simulink model "h16k_ver110_1080"  (R2012b)
settings: Solver=VariableStepDiscrete  SolverMode=SingleTasking  StartTime=0.0  StopTime=128000  RelTol=1e-3
undefined symbols (not defined in the file or in its folder): sfp
libraries: xbsIndex_r4 x3384, dspsigops x32, casper_library_misc x23, monroe_library x8, simulink x7, xps_library x6
(part 6 of 28)

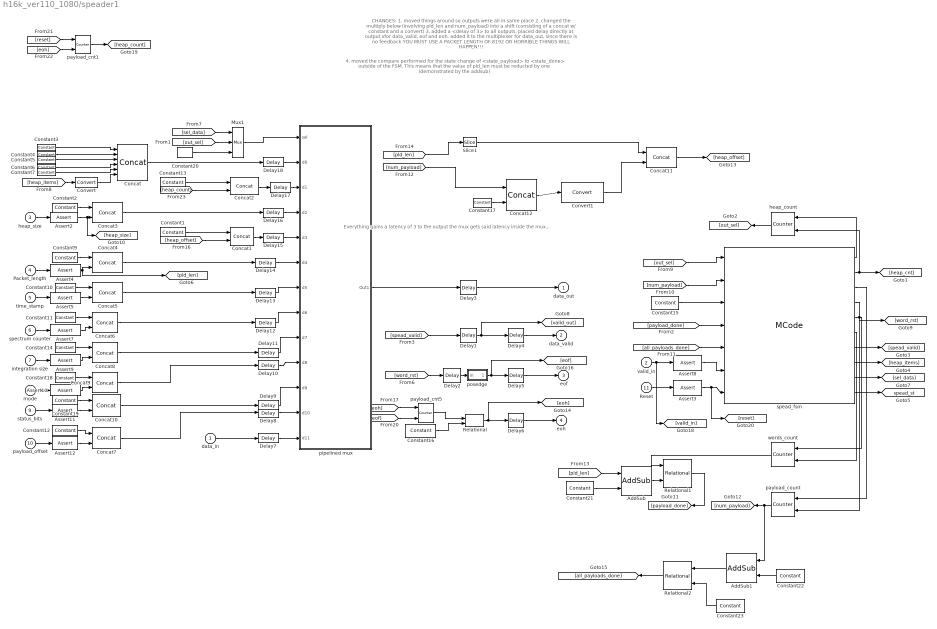
== system h16k_ver110_1080/speader1 ==
  note: Everything gains a latency of 3 to the output
      | the mux gets said latency inside the mux...
  note: CHANGES:
      | 1. moved things around so outputs were all in same place
      | 2. changed the multiply below (involving pld_len and num_payload) into a shift (consisting of a concat w/ constant and a convert)
      | 3. added a <delay of 3> to all outputs.  placed delay directly at output vfor data_valid, eof and eoh.  added it to the multiplexer for data_out, since there is no feedback
      |
      | YOU MUST USE A PACKET LENGTH OF 8192 OR HORRIBLE THINGS WILL HAPPEN!!!
  note: 4. moved the compare performed for the state change of <state_oayload> to <state_done> outside of the FSM.
      | This means that the value of pld_len must be reducted by one (demonstrated by the addsub)
  data_in : Inport
  valid_in : Inport  Port=2
  heap_size : Inport  Port=3
  Packet_length : Inport  Port=4
  time_stamp : Inport  Port=5
  spectrum counter : Inport  Port=6
  integration size : Inport  Port=7
  mode : Inport  Port=8
  status_bits : Inport  Port=9
  payload_offset : Inport  Port=10
  Reset : Inport  Port=11
  AddSub : xbsIndex_r4/AddSub  mode=Subtraction  use_carryin=off  use_carryout=off  en=off  latency=0  precision=User Defined  arith_type=Unsigned  n_bits=40  bin_pt=0  quantization=Truncate  overflow=Wrap  dbl_ovrd=off  use_behavioral_HDL=off  hw_selection=Fabric  pipelined=off  block_type=addsub
  AddSub1 : xbsIndex_r4/AddSub  mode=Addition  use_carryin=off  use_carryout=off  en=off  latency=1  precision=User Defined  arith_type=Unsigned  n_bits=8  bin_pt=0  quantization=Truncate  overflow=Wrap  dbl_ovrd=off  use_behavioral_HDL=off  hw_selection=Fabric  pipelined=off  block_type=addsub
  Assert{2,4..5,7,9..12} (8 alike) : xbsIndex_r4/Assert  assert_type=on  type_source=Explicitly  gui_display_data_type=Fixed-point  arith_type=Unsigned  n_bits=spead_lsw  bin_pt=0  preci_type=Single  exp_width=8  frac_width=24  assert_rate=off  rate_source=Explicitly  period=1  output_port=on  block_type=assert
      settings: block_version=11.4
  Assert3 : xbsIndex_r4/Assert  assert_type=on  type_source=Explicitly  gui_display_data_type=Fixed-point  arith_type=Boolean  n_bits=spead_lsw  bin_pt=0  preci_type=Single  exp_width=8  frac_width=24  assert_rate=on  rate_source=Explicitly  period=1  output_port=on  block_type=assert
      settings: block_version=11.4
  Assert8 : xbsIndex_r4/Assert  assert_type=on  type_source=Explicitly  gui_display_data_type=Fixed-point  arith_type=Boolean  n_bits=spead_lsw  bin_pt=0  preci_type=Single  exp_width=8  frac_width=24  assert_rate=on  rate_source=Explicitly  period=1  output_port=on  block_type=assert
      settings: block_version=11.4
  Concat : xbsIndex_r4/Concat  num_inputs=6  dbl_ovrd=off  block_type=concat
  Concat{1..12} (12 alike) : xbsIndex_r4/Concat  num_inputs=2  dbl_ovrd=off  block_type=concat
  Constant1 : xbsIndex_r4/Constant  const=8388608+3  gui_display_data_type=Fixed-point  arith_type=Unsigned  n_bits=spead_msw-spead_lsw  bin_pt=0  preci_type=Single  exp_width=8  frac_width=24  explicit_period=on  period=1  equ=P=C  opselect=C  inp2=PCIN>>17  opr=+  inp1=P  carry=CIN  dbl_ovrd=off  block_type=constant
      settings: block_version=11.4
  Constant10 : xbsIndex_r4/Constant  const=8388608+32  gui_display_data_type=Fixed-point  arith_type=Unsigned  n_bits=spead_msw-spead_lsw  bin_pt=0  preci_type=Single  exp_width=8  frac_width=24  explicit_period=on  period=1  equ=P=C  opselect=C  inp2=PCIN>>17  opr=+  inp1=P  carry=CIN  dbl_ovrd=off  block_type=constant
      settings: block_version=11.4
  Constant11 : xbsIndex_r4/Constant  const=8388608+33  gui_display_data_type=Fixed-point  arith_type=Unsigned  n_bits=spead_msw-spead_lsw  bin_pt=0  preci_type=Single  exp_width=8  frac_width=24  explicit_period=on  period=1  equ=P=C  opselect=C  inp2=PCIN>>17  opr=+  inp1=P  carry=CIN  dbl_ovrd=off  block_type=constant
      settings: block_version=11.4
  Constant12 : xbsIndex_r4/Constant  const=37  gui_display_data_type=Fixed-point  arith_type=Unsigned  n_bits=spead_msw-spead_lsw  bin_pt=0  preci_type=Single  exp_width=8  frac_width=24  explicit_period=on  period=1  equ=P=C  opselect=C  inp2=PCIN>>17  opr=+  inp1=P  carry=CIN  dbl_ovrd=off  block_type=constant
      settings: block_version=11.4
  Constant13 : xbsIndex_r4/Constant  const=8388608+1  gui_display_data_type=Fixed-point  arith_type=Unsigned  n_bits=spead_msw-spead_lsw  bin_pt=0  preci_type=Single  exp_width=8  frac_width=24  explicit_period=on  period=1  equ=P=C  opselect=C  inp2=PCIN>>17  opr=+  inp1=P  carry=CIN  dbl_ovrd=off  block_type=constant
      settings: block_version=11.4
  Constant14 : xbsIndex_r4/Constant  const=8388608+34  gui_display_data_type=Fixed-point  arith_type=Unsigned  n_bits=spead_msw-spead_lsw  bin_pt=0  preci_type=Single  exp_width=8  frac_width=24  explicit_period=on  period=1  equ=P=C  opselect=C  inp2=PCIN>>17  opr=+  inp1=P  carry=CIN  dbl_ovrd=off  block_type=constant
      settings: block_version=11.4
  Constant15 : xbsIndex_r4/Constant  const=num_items+5  gui_display_data_type=Fixed-point  arith_type=Unsigned  n_bits=8  bin_pt=0  preci_type=Single  exp_width=8  frac_width=24  explicit_period=on  period=1  equ=P=C  opselect=C  inp2=PCIN>>17  opr=+  inp1=P  carry=CIN  dbl_ovrd=off  block_type=constant
      settings: block_version=11.4
  Constant16 : xbsIndex_r4/Constant  const=num_payloads  gui_display_data_type=Fixed-point  arith_type=Unsigned  n_bits=16  bin_pt=0  preci_type=Single  exp_width=8  frac_width=24  explicit_period=on  period=1  equ=P=C  opselect=C  inp2=PCIN>>17  opr=+  inp1=P  carry=CIN  dbl_ovrd=off  block_type=constant
      settings: block_version=11.4
  Constant17 : xbsIndex_r4/Constant  const=0  gui_display_data_type=Fixed-point  arith_type=Unsigned  n_bits=13  bin_pt=0  preci_type=Single  exp_width=8  frac_width=24  explicit_period=on  period=1  equ=P=C  opselect=C  inp2=PCIN>>17  opr=+  inp1=P  carry=CIN  dbl_ovrd=off  block_type=constant
  Constant18 : xbsIndex_r4/Constant  const=8388608+35  gui_display_data_type=Fixed-point  arith_type=Unsigned  n_bits=spead_msw-spead_lsw  bin_pt=0  preci_type=Single  exp_width=8  frac_width=24  explicit_period=on  period=1  equ=P=C  opselect=C  inp2=PCIN>>17  opr=+  inp1=P  carry=CIN  dbl_ovrd=off  block_type=constant
      settings: block_version=11.4
  Constant19 : xbsIndex_r4/Constant  const=8388608+36  gui_display_data_type=Fixed-point  arith_type=Unsigned  n_bits=spead_msw-spead_lsw  bin_pt=0  preci_type=Single  exp_width=8  frac_width=24  explicit_period=on  period=1  equ=P=C  opselect=C  inp2=PCIN>>17  opr=+  inp1=P  carry=CIN  dbl_ovrd=off  block_type=constant
      settings: block_version=11.4
  Constant2 : xbsIndex_r4/Constant  const=8388608+2  gui_display_data_type=Fixed-point  arith_type=Unsigned  n_bits=spead_msw-spead_lsw  bin_pt=0  preci_type=Single  exp_width=8  frac_width=24  explicit_period=on  period=1  equ=P=C  opselect=C  inp2=PCIN>>17  opr=+  inp1=P  carry=CIN  dbl_ovrd=off  block_type=constant
      settings: block_version=11.4
  Constant20 : xbsIndex_r4/Constant  const=num_items+5  gui_display_data_type=Fixed-point  arith_type=Unsigned  n_bits=4  bin_pt=0  preci_type=Single  exp_width=8  frac_width=24  explicit_period=on  period=1  equ=P=C  opselect=C  inp2=PCIN>>17  opr=+  inp1=P  carry=CIN  dbl_ovrd=off  block_type=constant
      settings: block_version=11.4
  Constant21 : xbsIndex_r4/Constant  const=8  gui_display_data_type=Fixed-point  arith_type=Unsigned  n_bits=4  bin_pt=0  preci_type=Single  exp_width=8  frac_width=24  explicit_period=on  period=1  equ=P=C  opselect=C  inp2=PCIN>>17  opr=+  inp1=P  carry=CIN  dbl_ovrd=off  block_type=constant
      settings: block_version=11.4
  Constant22 : xbsIndex_r4/Constant  const=1  gui_display_data_type=Fixed-point  arith_type=Unsigned  n_bits=1  bin_pt=0  preci_type=Single  exp_width=8  frac_width=24  explicit_period=on  period=1  equ=P=C  opselect=C  inp2=PCIN>>17  opr=+  inp1=P  carry=CIN  dbl_ovrd=off  block_type=constant
      settings: block_version=11.4
  Constant23 : xbsIndex_r4/Constant  const=num_payloads  gui_display_data_type=Fixed-point  arith_type=Unsigned  n_bits=8  bin_pt=0  preci_type=Single  exp_width=8  frac_width=24  explicit_period=on  period=1  equ=P=C  opselect=C  inp2=PCIN>>17  opr=+  inp1=P  carry=CIN  dbl_ovrd=off  block_type=constant
      settings: block_version=11.4
  Constant3 : xbsIndex_r4/Constant  const=83  gui_display_data_type=Fixed-point  arith_type=Unsigned  n_bits=8  bin_pt=0  preci_type=Single  exp_width=8  frac_width=24  explicit_period=on  period=1  equ=P=C  opselect=C  inp2=PCIN>>17  opr=+  inp1=P  carry=CIN  dbl_ovrd=off  block_type=constant
      settings: block_version=11.4
  Constant4 : xbsIndex_r4/Constant  const=4  gui_display_data_type=Fixed-point  arith_type=Unsigned  n_bits=8  bin_pt=0  preci_type=Single  exp_width=8  frac_width=24  explicit_period=on  period=1  equ=P=C  opselect=C  inp2=PCIN>>17  opr=+  inp1=P  carry=CIN  dbl_ovrd=off  block_type=constant
      settings: block_version=11.4
  Constant5 : xbsIndex_r4/Constant  const=3  gui_display_data_type=Fixed-point  arith_type=Unsigned  n_bits=8  bin_pt=0  preci_type=Single  exp_width=8  frac_width=24  explicit_period=on  period=1  equ=P=C  opselect=C  inp2=PCIN>>17  opr=+  inp1=P  carry=CIN  dbl_ovrd=off  block_type=constant
      settings: block_version=11.4
  Constant6 : xbsIndex_r4/Constant  const=5  gui_display_data_type=Fixed-point  arith_type=Unsigned  n_bits=8  bin_pt=0  preci_type=Single  exp_width=8  frac_width=24  explicit_period=on  period=1  equ=P=C  opselect=C  inp2=PCIN>>17  opr=+  inp1=P  carry=CIN  dbl_ovrd=off  block_type=constant
      settings: block_version=11.4
  Constant7 : xbsIndex_r4/Constant  const=0  gui_display_data_type=Fixed-point  arith_type=Unsigned  n_bits=16  bin_pt=0  preci_type=Single  exp_width=8  frac_width=24  explicit_period=on  period=1  equ=P=C  opselect=C  inp2=PCIN>>17  opr=+  inp1=P  carry=CIN  dbl_ovrd=off  block_type=constant
      settings: block_version=11.4
  Constant9 : xbsIndex_r4/Constant  const=8388608+4  gui_display_data_type=Fixed-point  arith_type=Unsigned  n_bits=spead_msw-spead_lsw  bin_pt=0  preci_type=Single  exp_width=8  frac_width=24  explicit_period=on  period=1  equ=P=C  opselect=C  inp2=PCIN>>17  opr=+  inp1=P  carry=CIN  dbl_ovrd=off  block_type=constant
      settings: block_version=11.4
  Convert : xbsIndex_r4/Convert  gui_display_data_type=Fixed-point  arith_type=Unsigned  n_bits=16  bin_pt=0  float_type=Single  exp_bits=8  fraction_bits=24  quantization=Truncate  overflow=Wrap  en=off  latency=0  dbl_ovrd=off  pipeline=off  block_type=convert
      settings: block_version=11.4
  Convert1 : xbsIndex_r4/Convert  gui_display_data_type=Fixed-point  arith_type=Unsigned  n_bits=25  bin_pt=0  float_type=Single  exp_bits=8  fraction_bits=24  quantization=Truncate  overflow=Wrap  en=off  latency=3  dbl_ovrd=off  pipeline=off  block_type=convert
  Delay{1,3,7..18} (14 alike) : xbsIndex_r4/Delay  rst=off  infoeditControl=Selection of Reset will increase slice count due to use of real FFs and instead of SRLs  en=off  latency=1  dbl_ovrd=off  reg_retiming=on  block_type=delay
      settings: block_version=11.4
  Delay2 : xbsIndex_r4/Delay  rst=off  infoeditControl=Selection of Reset will increase slice count due to use of real FFs and instead of SRLs  en=off  latency=0  dbl_ovrd=off  reg_retiming=on  block_type=delay
      settings: block_version=11.4
  Delay4 : xbsIndex_r4/Delay  rst=off  infoeditControl=Selection of Reset will increase slice count due to use of real FFs and instead of SRLs  en=off  latency=3  dbl_ovrd=off  reg_retiming=on  block_type=delay
      settings: block_version=11.4
  Delay5 : xbsIndex_r4/Delay  rst=off  infoeditControl=Selection of Reset will increase slice count due to use of real FFs and instead of SRLs  en=off  latency=3  dbl_ovrd=off  reg_retiming=on  block_type=delay
      settings: block_version=11.4
  Delay6 : xbsIndex_r4/Delay  rst=off  infoeditControl=Selection of Reset will increase slice count due to use of real FFs and instead of SRLs  en=off  latency=3  dbl_ovrd=off  reg_retiming=on  block_type=delay
      settings: block_version=11.4
  Mux1 : xbsIndex_r4/Mux  inputs=2  en=off  latency=1  precision=Full  arith_type="Signed  (2's comp)"  n_bits=8  bin_pt=2  quantization=Truncate  overflow=Wrap  dbl_ovrd=off  block_type=mux
      settings: block_version=11.4
  Relational : xbsIndex_r4/Relational  mode=a=b  en=off  latency=0  dbl_ovrd=off  block_type=relational
  Relational1 : xbsIndex_r4/Relational  mode=a=b  en=off  latency=1  dbl_ovrd=off  block_type=relational
  Relational2 : xbsIndex_r4/Relational  mode=a=b  en=off  latency=1  dbl_ovrd=off  block_type=relational
  Slice1 : xbsIndex_r4/Slice  nbits=15  boolean_output=off  mode=Upper Bit Location + Width  bit1=0  base1=MSB of Input  bit0=0  base0=LSB of Input  dbl_ovrd=off  block_type=slice
      settings: block_version=10.1.3
  heap_count : xbsIndex_r4/Counter  cnt_type=Free Running  cnt_to=Inf  operation=Up  start_count=0  cnt_by_val=1  arith_type=Unsigned  n_bits=4  bin_pt=0  load_pin=off  rst=on  en=on  explicit_period=on  period=1  dbl_ovrd=off  use_behavioral_HDL=off  implementation=Fabric  block_type=counter
      settings: block_version=11.4
  payload_cnt1 : xbsIndex_r4/Counter  cnt_type=Free Running  cnt_to=0  operation=Up  start_count=1024  cnt_by_val=1  arith_type=Unsigned  n_bits=40  bin_pt=0  load_pin=off  rst=on  en=on  explicit_period=on  period=1  dbl_ovrd=off  use_behavioral_HDL=off  implementation=Fabric  use_rpm=on  block_type=counter
      settings: xl_area=[0, 0, 0, 0, 0, 0, 0]
  payload_cnt5 : xbsIndex_r4/Counter  cnt_type=Free Running  cnt_to=0  operation=Up  start_count=0  cnt_by_val=1  arith_type=Unsigned  n_bits=16  bin_pt=0  load_pin=off  rst=on  en=on  explicit_period=on  period=1  dbl_ovrd=off  use_behavioral_HDL=off  implementation=Fabric  use_rpm=on  block_type=counter
      settings: xl_area=[0, 0, 0, 0, 0, 0, 0]
  payload_count : xbsIndex_r4/Counter  cnt_type=Free Running  cnt_to=Inf  operation=Up  start_count=0  cnt_by_val=1  arith_type=Unsigned  n_bits=8  bin_pt=0  load_pin=off  rst=on  en=on  explicit_period=on  period=1  dbl_ovrd=off  use_behavioral_HDL=off  implementation=Fabric  block_type=counter
      settings: block_version=11.4
  pipelined mux : Subsystem
  posedge : Subsystem  AncestorBlock=casper_library_misc/edge_detect  mask(edge_detect){edge=Rising, polarity=Active High, x_in=[0 0.08 0.08 0.16 0.16 0.24 0.24 0.32 0.32 0.4], y_in=[-1 -1  1  1  1  1  1  1  1  1], x_out=[0.6 0.68 0.68 0.76 0.76 0.84 0.84 0.92 0.92 1], y_out=[-1 -1  1  1 -1 -1 -1 -1 -1 -1]}
      mask prompts: edge "Edge Type"; polarity "Output Polarity"; x_in "Input X Positions"; y_in "Input Y Positions"; x_out "Output X Positions"; y_out "Output Y Positions"
      mask help: Output is active for one-cycle after each edge of the specified type (i.e. rising, falling or both).
      mask init: same as h16k_ver110_1080/edge_detect
      settings: AttributesFormatString=|
      | rising edges
      | active high
      mask Help: Output is active for one-cycle after each edge of the specified type (i.e. rising, falling, or both).  Latency is zero.
      mask TypeOptions edge: Rising | Falling | Both
      mask TypeOptions polarity: Active High | Active Low
      mask Display:
      | plot(x_in_num,0.5+y_in_num*0.2);
      | plot(x_out_num,0.5+y_out_num*0.2);
  spead_fsm : xbsIndex_r4/MCode  mfname=spead_fsm_v2  explicit_period=on  period=1  inputsTable={'boundInpExpr'=>['','','','5','','','',''],'inputs'=>['head_count','num_payload_sent','total_header_len','min_header_len','payload_done','all_payloads_done','data_valid_in','rst']}  outputsTable={'outputs'=>['head_count_rst','head_count_en','num_payload_rst','num_payload_en','words_sent_rst','words_sent_en','tge_valid','heap_elements','select_data','st'],'suppressOut'=>['off','off','off','off','off','off','off','off','off','off']}  dbl_ovrd=off  enable_stdout=off  enable_debug=off  suppress_output=on  defparams={'min_header_len',5}  hide_port_list={}  block_type=mcode
      settings: block_version=11.4
  words_count : xbsIndex_r4/Counter  cnt_type=Free Running  cnt_to=Inf  operation=Up  start_count=0  cnt_by_val=8  arith_type=Unsigned  n_bits=15  bin_pt=0  load_pin=off  rst=on  en=on  explicit_period=on  period=1  dbl_ovrd=off  use_behavioral_HDL=off  implementation=Fabric  block_type=counter
      settings: block_version=11.4
  data_out : Outport
  data_valid : Outport  Port=2
  eof : Outport  Port=3
  eoh : Outport  Port=4
  tag scope: spead_st=global
  wires:
  Slice1/1 -> Concat11/1
  Concat11/1 -> [heap_offset]
  [eoh] -> payload_cnt1/2
  [reset] -> payload_cnt1/1
  payload_cnt1/1 -> [heap_count]
  payload_cnt5/1 -> Relational/1
  Constant16/1 -> Relational/2
  Relational/1 -> [eoh], Delay6/1
  [eof] -> payload_cnt5/2
  [eoh] -> payload_cnt5/1
  [sel_data] -> Mux1/1
  [out_sel] -> Mux1/2
  pipelined mux/1(Out1) -> Delay3/1
  [pld_len] -> Slice1/1
  [num_payload] -> Concat12/1
  Delay2/1 -> posedge/1(in)
  Constant15/1 -> spead_fsm/3
  [all_payloads_done] -> spead_fsm/5
  Assert8/1 -> spead_fsm/6
  Assert3/1 -> [reset], spead_fsm/7
  [word_rst] -> Delay2/1
  posedge/1(out) -> [eof], Delay5/1
  [num_payload] -> spead_fsm/2
  [out_sel] -> spead_fsm/1
  heap_count/1 -> [out_sel]
  payload_count/1 -> [num_payload], AddSub1/1
  Convert/1 -> Concat/6
  [heap_items] -> Convert/1
  spead_fsm/9 -> [sel_data]
  spead_fsm/10 -> [spead_st]
  Mux1/1 -> pipelined mux/1(sel)
  Constant20/1 -> Mux1/3
  Reset/1 -> Assert3/1
  [heap_offset] -> Concat1/2
  valid_in/1 -> [valid_in], Assert8/1
  spead_fsm/8 -> [heap_items]
  spead_fsm/7 -> [spead_valid]
  spead_fsm/2 -> [heap_cnt], heap_count/2
  spead_fsm/1 -> heap_count/1
  spead_fsm/4 -> [word_rst], payload_count/2
  spead_fsm/3 -> payload_count/1
  spead_fsm/6 -> words_count/2
  spead_fsm/5 -> words_count/1
  Concat8/1 -> Delay11/1
  Constant14/1 -> Concat8/1
  Assert9/1 -> Concat8/2
  integration size/1 -> Assert9/1
  Concat5/1 -> Delay13/1
  Concat6/1 -> Delay12/1
  Constant11/1 -> Concat6/1
  Assert7/1 -> Concat6/2
  spectrum counter/1 -> Assert7/1
  Concat9/1 -> Delay10/1
  Concat10/1 -> Delay9/1
  Concat7/1 -> Delay8/1
  Concat1/1 -> Delay15/1
  Constant1/1 -> Concat1/1
  Delay1/1 -> [valid_out], Delay4/1
  Packet_length/1 -> Assert4/1
  [spead_valid] -> Delay1/1
  Concat2/1 -> Delay17/1
  Assert5/1 -> Concat5/2
  Assert4/1 -> [pld_len], Concat4/2
  Assert2/1 -> [heap_size], Concat3/2
  [heap_count] -> Concat2/2
  heap_size/1 -> Assert2/1
  time_stamp/1 -> Assert5/1
  data_in/1 -> Delay7/1
  Constant10/1 -> Concat5/1
  Constant12/1 -> Concat7/1
  Constant13/1 -> Concat2/1
  Constant2/1 -> Concat3/1
  Constant3/1 -> Concat/1
  Constant4/1 -> Concat/2
  Constant5/1 -> Concat/3
  Constant6/1 -> Concat/4
  Constant7/1 -> Concat/5
  Constant9/1 -> Concat4/1
  Concat/1 -> Delay18/1
  Concat3/1 -> Delay16/1
  Concat4/1 -> Delay14/1
  Constant18/1 -> Concat9/1
  mode/1 -> Assert10/1
  Assert10/1 -> Concat9/2
  Constant19/1 -> Concat10/1
  status_bits/1 -> Assert11/1
  Assert11/1 -> Concat10/2
  payload_offset/1 -> Assert12/1
  Assert12/1 -> Concat7/2
  Delay3/1 -> data_out/1
  Delay4/1 -> data_valid/1
  Delay5/1 -> eof/1
  Delay6/1 -> eoh/1
  Constant17/1 -> Concat12/2
  Concat12/1 -> Convert1/1
  Convert1/1 -> Concat11/2
  [pld_len] -> AddSub/1
  Constant21/1 -> AddSub/2
  AddSub/1 -> Relational1/2
  Relational1/1 -> [payload_done]
  words_count/1 -> Relational1/1
  Delay7/1 -> pipelined mux/13(d11)
  Delay8/1 -> pipelined mux/12(d10)
  Delay9/1 -> pipelined mux/11(d9)
  Delay10/1 -> pipelined mux/10(d8)
  Delay11/1 -> pipelined mux/9(d7)
  Delay12/1 -> pipelined mux/8(d6)
  Delay13/1 -> pipelined mux/7(d5)
  Delay14/1 -> pipelined mux/6(d4)
  Delay15/1 -> pipelined mux/5(d3)
  Delay16/1 -> pipelined mux/4(d2)
  Delay17/1 -> pipelined mux/3(d1)
  Delay18/1 -> pipelined mux/2(d0)
  Constant22/1 -> AddSub1/2
  AddSub1/1 -> Relational2/1
  Constant23/1 -> Relational2/2
  Relational2/1 -> [all_payloads_done]
  [payload_done] -> spead_fsm/4
